simulink model "PID_TN"  (Simulink 7.3)
settings: Solver=ode5  StartTime=0.0  StopTime=80  FixedStep=0.01  RelTol=1e-3
StopFcn:
  | subplot(211);
  | plot(Data.time,Data.signals(1).values(:,1),'r',Data.time,Data.signals(1).values(:,2),'b')
  | subplot(212);
  | plot(Data.time,Data.signals(2).values(:,1),'b')
values from neighbouring files (symbols this model uses):
  a1 = -p-conj(p)    [ARMA_vs_Correlogram.m]    (also in AR_vs_Correlogram.m; tn_nn1.m = 1; tn_nn2.m = 1./p1)
undefined symbols (not defined in the file or in its folder): a0, k
libraries: simulink x1
settings Model: Creator=Minh-Map-Vu  LastModifiedBy=nthuy
settings DataIOCC: SignalLoggingName=sigsOut
settings DebuggingCC: SaveWithParameterizedLinksMsg=none  SignalResolutionControl=TryResolveAllWithWarning  SolverPrmCheckMsg=none  MultiTaskDSMMsg=warning  MultiTaskCondExecSysMsg=none  StrictBusMsg=None
settings HardwareCC: TargetEndianess=LittleEndian  TargetHWDeviceType=MATLAB Host  ProdEqTarget=off
settings RTWCC: IncludeERTFirstTime=on

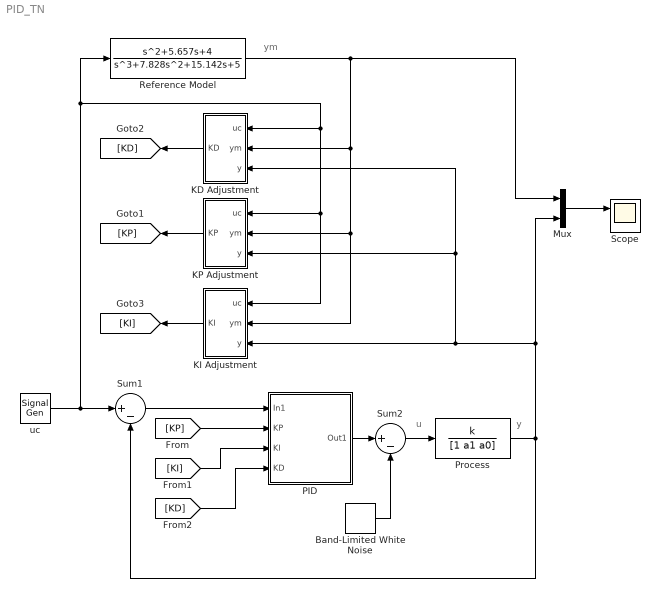
== system PID_TN ==
  note: ym
  note: u
  note: y
  Band-Limited White Noise : simulink/Sources/Band-Limited White Noise  SystemSampleTime=-1  Cov=[0.1]  Ts=0.01  seed=[23341]
  "KD Adjustment " : Subsystem
  KI Adjustment : Subsystem
  KP Adjustment : Subsystem
  Mux : Mux  Inputs=2
  PID : Subsystem
  Process : TransferFcn  Numerator=k  Denominator=[1 a1 a0]
  Reference Model : TransferFcn  Numerator=[1 5.657 4]  Denominator=[1 7.828 15.142 5]
  Scope : Scope  NumInputPorts=2
      settings: TimeRange=100  YMin=-1.2~-5  YMax=1.2~5  SaveName=Data
  Sum1 : Sum  Inputs=|+-  SaturateOnIntegerOverflow=on
  Sum2 : Sum  Inputs=|+-  SaturateOnIntegerOverflow=on
  uc : SignalGenerator  WaveForm=square  Frequency=1/20
  wires:
  uc/1 -> Sum1/1, Reference Model/1, "KD Adjustment "/1(uc), KI Adjustment/1(uc), KP Adjustment/1(uc)
  Reference Model/1 -> Mux/1, KI Adjustment/2(ym), KP Adjustment/2(ym), "KD Adjustment "/2(ym)
  Process/1 -> Sum1/2, Mux/2, KI Adjustment/3(y), "KD Adjustment "/3(y), KP Adjustment/3(y)
  Mux/1 -> Scope/1
  Sum1/1 -> PID/1(In1)
  "KD Adjustment "/1(KD) -> [KD]
  KP Adjustment/1(KP) -> [KP]
  KI Adjustment/1(KI) -> [KI]
  [KP] -> PID/2(KP)
  [KI] -> PID/3(KI)
  [KD] -> PID/4(KD)
  PID/1(Out1) -> Sum2/1
  Sum2/1 -> Process/1
  Band-Limited White Noise/1 -> Sum2/2

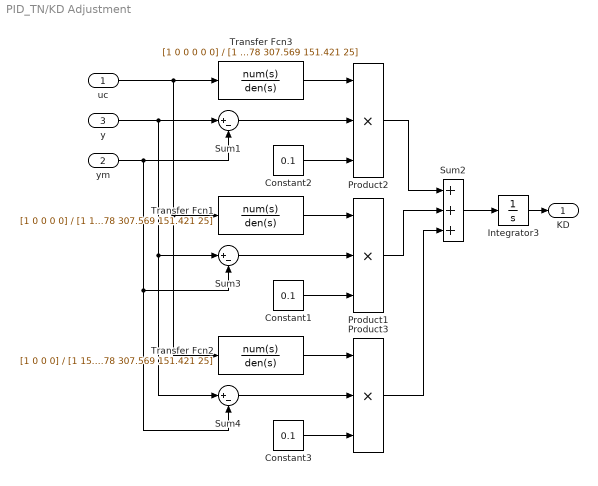
== system PID_TN/KD Adjustment  ==
  uc : Inport  OutDataType=fixdt(1, 16)  OutScaling=2^0
  ym : Inport  Port=2  OutDataType=fixdt(1, 16)  OutScaling=2^0
  y : Inport  Port=3  OutDataType=fixdt(1, 16)  OutScaling=2^0
  Constant1 : Constant  Value=0.1  OutDataType=fixdt(1, 16)  OutScaling=2^0
  Constant2 : Constant  Value=0.1  OutDataType=fixdt(1, 16)  OutScaling=2^0
  Constant3 : Constant  Value=0.1  OutDataType=fixdt(1, 16)  OutScaling=2^0
  Integrator3 : Integrator
  Product1 : Product  Inputs=3  SaturateOnIntegerOverflow=on  OutDataTypeStr=Inherit: Same as first input
  Product2 : Product  Inputs=3  SaturateOnIntegerOverflow=on  OutDataTypeStr=Inherit: Same as first input
  Product3 : Product  Inputs=3  SaturateOnIntegerOverflow=on  OutDataTypeStr=Inherit: Same as first input
  Sum1 : Sum  Inputs=|+-  OutDataType=fixdt(1, 16)  OutScaling=2^0
  Sum2 : Sum  Inputs=+++  SaturateOnIntegerOverflow=on
  Sum3 : Sum  Inputs=|+-  OutDataType=fixdt(1, 16)  OutScaling=2^0
  Sum4 : Sum  Inputs=|+-  OutDataType=fixdt(1, 16)  OutScaling=2^0
  Transfer Fcn1 : TransferFcn  Numerator=[1 0 0 0 0]  Denominator=[1 15.657 91.569 247.078 307.569 151.421 25]
  Transfer Fcn2 : TransferFcn  Numerator=[1 0 0 0]  Denominator=[1 15.657 91.569 247.078 307.569 151.421 25]
  Transfer Fcn3 : TransferFcn  Numerator=[1 0 0 0 0 0]  Denominator=[1 15.657 91.569 247.078 307.569 151.421 25]
  KD : Outport
  wires:
  y/1 -> Sum1/1, Sum3/1, Sum4/1
  ym/1 -> Sum1/2, Sum3/2, Sum4/2
  Transfer Fcn3/1 -> Product2/1
  uc/1 -> Transfer Fcn3/1, Transfer Fcn1/1, Transfer Fcn2/1
  Sum1/1 -> Product2/2
  Constant2/1 -> Product2/3
  Integrator3/1 -> KD/1
  Product2/1 -> Sum2/1
  Sum2/1 -> Integrator3/1
  Transfer Fcn1/1 -> Product1/1
  Sum3/1 -> Product1/2
  Constant1/1 -> Product1/3
  Transfer Fcn2/1 -> Product3/1
  Sum4/1 -> Product3/2
  Constant3/1 -> Product3/3
  Product1/1 -> Sum2/2
  Product3/1 -> Sum2/3

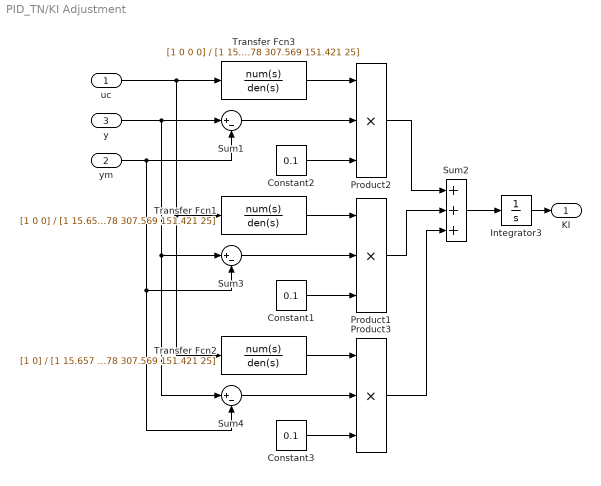
== system PID_TN/KI Adjustment ==
  uc : Inport  OutDataType=fixdt(1, 16)  OutScaling=2^0
  ym : Inport  Port=2  OutDataType=fixdt(1, 16)  OutScaling=2^0
  y : Inport  Port=3  OutDataType=fixdt(1, 16)  OutScaling=2^0
  Constant1 : Constant  Value=0.1  OutDataType=fixdt(1, 16)  OutScaling=2^0
  Constant2 : Constant  Value=0.1  OutDataType=fixdt(1, 16)  OutScaling=2^0
  Constant3 : Constant  Value=0.1  OutDataType=fixdt(1, 16)  OutScaling=2^0
  Integrator3 : Integrator
  Product1 : Product  Inputs=3  SaturateOnIntegerOverflow=on  OutDataTypeStr=Inherit: Same as first input
  Product2 : Product  Inputs=3  SaturateOnIntegerOverflow=on  OutDataTypeStr=Inherit: Same as first input
  Product3 : Product  Inputs=3  SaturateOnIntegerOverflow=on  OutDataTypeStr=Inherit: Same as first input
  Sum1 : Sum  Inputs=|+-  OutDataType=fixdt(1, 16)  OutScaling=2^0
  Sum2 : Sum  Inputs=+++  SaturateOnIntegerOverflow=on
  Sum3 : Sum  Inputs=|+-  OutDataType=fixdt(1, 16)  OutScaling=2^0
  Sum4 : Sum  Inputs=|+-  OutDataType=fixdt(1, 16)  OutScaling=2^0
  Transfer Fcn1 : TransferFcn  Numerator=[1 0 0]  Denominator=[1 15.657 91.569 247.078 307.569 151.421 25]
  Transfer Fcn2 : TransferFcn  Numerator=[1 0]  Denominator=[1 15.657 91.569 247.078 307.569 151.421 25]
  Transfer Fcn3 : TransferFcn  Numerator=[1 0 0 0]  Denominator=[1 15.657 91.569 247.078 307.569 151.421 25]
  KI : Outport
  wires:
  y/1 -> Sum1/1, Sum3/1, Sum4/1
  ym/1 -> Sum1/2, Sum3/2, Sum4/2
  Transfer Fcn3/1 -> Product2/1
  uc/1 -> Transfer Fcn3/1, Transfer Fcn1/1, Transfer Fcn2/1
  Sum1/1 -> Product2/2
  Constant2/1 -> Product2/3
  Integrator3/1 -> KI/1
  Product2/1 -> Sum2/1
  Sum2/1 -> Integrator3/1
  Transfer Fcn1/1 -> Product1/1
  Sum3/1 -> Product1/2
  Constant1/1 -> Product1/3
  Transfer Fcn2/1 -> Product3/1
  Sum4/1 -> Product3/2
  Constant3/1 -> Product3/3
  Product1/1 -> Sum2/2
  Product3/1 -> Sum2/3

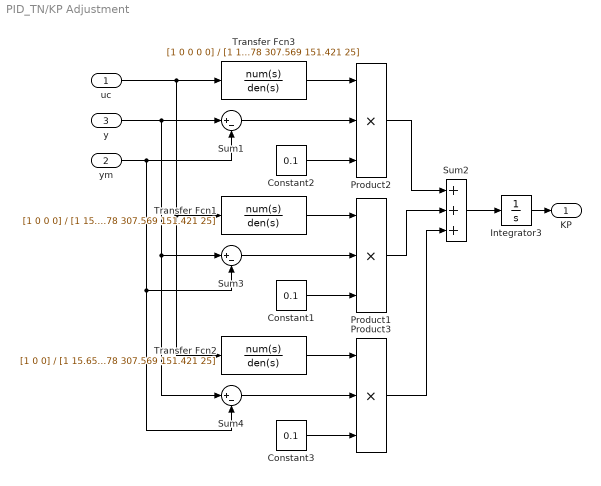
== system PID_TN/KP Adjustment ==
  uc : Inport  OutDataType=fixdt(1, 16)  OutScaling=2^0
  ym : Inport  Port=2  OutDataType=fixdt(1, 16)  OutScaling=2^0
  y : Inport  Port=3  OutDataType=fixdt(1, 16)  OutScaling=2^0
  Constant1 : Constant  Value=0.1  OutDataType=fixdt(1, 16)  OutScaling=2^0
  Constant2 : Constant  Value=0.1  OutDataType=fixdt(1, 16)  OutScaling=2^0
  Constant3 : Constant  Value=0.1  OutDataType=fixdt(1, 16)  OutScaling=2^0
  Integrator3 : Integrator
  Product1 : Product  Inputs=3  SaturateOnIntegerOverflow=on  OutDataTypeStr=Inherit: Same as first input
  Product2 : Product  Inputs=3  SaturateOnIntegerOverflow=on  OutDataTypeStr=Inherit: Same as first input
  Product3 : Product  Inputs=3  SaturateOnIntegerOverflow=on  OutDataTypeStr=Inherit: Same as first input
  Sum1 : Sum  Inputs=|+-  OutDataType=fixdt(1, 16)  OutScaling=2^0
  Sum2 : Sum  Inputs=+++  SaturateOnIntegerOverflow=on
  Sum3 : Sum  Inputs=|+-  OutDataType=fixdt(1, 16)  OutScaling=2^0
  Sum4 : Sum  Inputs=|+-  OutDataType=fixdt(1, 16)  OutScaling=2^0
  Transfer Fcn1 : TransferFcn  Numerator=[1 0 0 0]  Denominator=[1 15.657 91.569 247.078 307.569 151.421 25]
  Transfer Fcn2 : TransferFcn  Numerator=[1 0 0]  Denominator=[1 15.657 91.569 247.078 307.569 151.421 25]
  Transfer Fcn3 : TransferFcn  Numerator=[1 0 0 0 0]  Denominator=[1 15.657 91.569 247.078 307.569 151.421 25]
  KP : Outport
  wires:
  Product3/1 -> Sum2/3
  Product1/1 -> Sum2/2
  Constant3/1 -> Product3/3
  Sum4/1 -> Product3/2
  Transfer Fcn2/1 -> Product3/1
  Constant1/1 -> Product1/3
  Sum3/1 -> Product1/2
  Transfer Fcn1/1 -> Product1/1
  Sum2/1 -> Integrator3/1
  Product2/1 -> Sum2/1
  Integrator3/1 -> KP/1
  Constant2/1 -> Product2/3
  Sum1/1 -> Product2/2
  uc/1 -> Transfer Fcn2/1, Transfer Fcn1/1, Transfer Fcn3/1
  Transfer Fcn3/1 -> Product2/1
  ym/1 -> Sum4/2, Sum3/2, Sum1/2
  y/1 -> Sum4/1, Sum3/1, Sum1/1

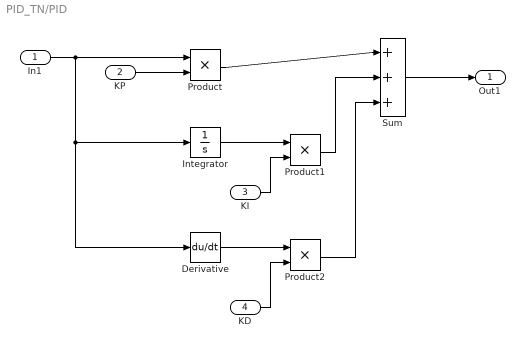
== system PID_TN/PID ==
  In1 : Inport
  KP : Inport  Port=2
  KI : Inport  Port=3
  KD : Inport  Port=4
  Derivative : Derivative
  Integrator : Integrator
  Product : Product  OutDataType=fixdt(1, 16)  OutScaling=2^0  RndMeth=Zero
  Product1 : Product  OutDataType=fixdt(1, 16)  OutScaling=2^0  RndMeth=Zero
  Product2 : Product  OutDataType=fixdt(1, 16)  OutScaling=2^0  RndMeth=Zero
  Sum : Sum  Inputs=|+++  OutDataType=fixdt(1, 16)  OutScaling=2^0
  Out1 : Outport
  wires:
  In1/1 -> Product/1, Integrator/1, Derivative/1
  KP/1 -> Product/2
  Integrator/1 -> Product1/1
  Derivative/1 -> Product2/1
  KI/1 -> Product1/2
  KD/1 -> Product2/2
  Product/1 -> Sum/1
  Product1/1 -> Sum/2
  Product2/1 -> Sum/3
  Sum/1 -> Out1/1
